simulink model "single_phase_deneme"  (R2018a)
settings: Solver=FixedStepDiscrete  StartTime=0.0  StopTime=0.07  FixedStep=5e-6  RelTol=1e-4  EnableMultiTasking=on
PreLoadFcn:
  | Ts=5e-6;
InitFcn:
  | Ts=5e-6;
libraries: powerlib x18, powerlib_meascontrol x2
Description:
  | Copyright 2008-2018 The MathWorks, Inc.
settings Model: Creator=MathWorks  LastModifiedBy=enes_
settings SolverCC: SolverResetMethod=Robust
settings DataIOCC: SaveOutput=off  SignalLogging=off  DSMLogging=off  SaveTime=off
settings OptimizationCC: LifeSpan=inf
settings DebuggingCC: ReadBeforeWriteMsg=DisableAll  WriteAfterWriteMsg=DisableAll  WriteAfterReadMsg=DisableAll  MultiTaskDSMMsg=none  SFUnexpectedBacktrackingDiag=warning  SFNoUnconditionalDefaultTransitionDiag=warning  SFExecutionAtInitializationDiag=none
settings ModelReferenceCC: UpdateModelReferenceTargets=IfOutOfDate
settings SFSimCC: SFSimEcho=off
settings CodeAppCC: StateflowObjectComments=on
settings GRTTargetCC: TargetLangStandard=C89/C90 (ANSI)  GeneratePreprocessorConditionals=Disable all
settings ConfigComp: CovMetricSettings=dw  CovHtmlReporting=on  CovSaveCumulativeToWorkspaceVar=on  CovSaveSingleToWorkspaceVar=on  CovExternalEMLEnable=off
settings SimscapeCC: SimscapeNormalizeSystem=off  SimscapeNominalValues={1, 'bar'; 1, 'cm^3/s'; 1, 'bar*kg/s'; 1, 'kJ/kg'; 1, 'kW'; }

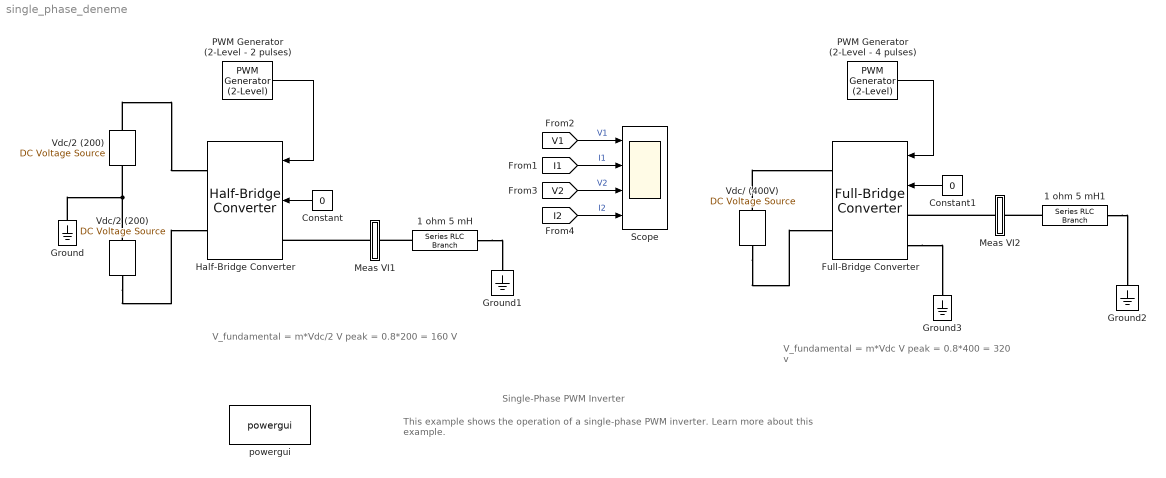
== system single_phase_deneme ==
  note: V_fundamental = m*Vdc/2 V peak
      | = 0.8*200
      | = 160 V
  note: Single-Phase PWM Inverter
  note: This example shows the operation of a single-phase PWM inverter.
      |
      | Learn more about this example.
  note: V_fundamental = m*Vdc V peak
      | = 0.8*400
      | = 320 v
  1 ohm 5 mH : powerlib/Elements/Series RLC Branch  LConnTagsString=__new0  RConnTagsString=__new0  BranchType=RL  Resistance=1  Inductance=5e-3  SetiL0=off  InitialCurrent=0  Capacitance=400e-6  Setx0=off  InitialVoltage=0  Measurements=None
  1 ohm 5 mH1 : powerlib/Elements/Series RLC Branch  LConnTagsString=__new0  RConnTagsString=__new0  BranchType=RL  Resistance=1  Inductance=5e-3  SetiL0=off  InitialCurrent=0  Capacitance=400e-6  Setx0=off  InitialVoltage=0  Measurements=None
  Constant : Constant  Value=0
  Constant1 : Constant  Value=0
  Full-Bridge Converter : powerlib/Power Electronics/Full-Bridge Converter  ModelType=Switching devices  Ron=1e-3  Rs=1e6  Cs=inf  Vforward=[0,0]  Ron_Diode=1e-3  Rs_Diode=1e6  Cs_Diode=inf  Vf_Diode=1e-3  Rs_CurrentSource=inf
      settings: SourceProductName=Simscape Power Systems  SourceProductBaseCode=PS
  Ground{,1..3} (4 alike) : powerlib/Elements/Ground  LConnTagsString=a
  Half-Bridge Converter : powerlib/Power Electronics/Half-Bridge Converter  ModelType=Switching devices  Ron=1e-3  Rs=1e6  Cs=inf  Vforward=[0,0]  Ron_Diode=1e-3  Rs_Diode=1e6  Cs_Diode=inf  Vf_Diode=1e-3  Rs_CurrentSource=inf
      settings: SourceProductName=Simscape Power Systems  SourceProductBaseCode=PS
  Meas VI1 : Subsystem
  Meas VI2 : Subsystem
  PWM Generator (2-Level - 2 pulses) : powerlib_meascontrol/Pulse & Signal Generators/PWM Generator (2-Level)  ModulatorType=Single-phase half-bridge (2 pulses)  ModulatorMode=Unsynchronized  Fc=27*60  Pc=90  nF=27  MinMax="[ -1  1 ]"  SamplingTechnique=Natural  ModulatingSignals=on  m=0.8  Freq=60  Phase=0  Ts=5e-6  ShowCarrierOutport=off
      settings: SourceProductName=Simscape Power Systems
  PWM Generator (2-Level - 4 pulses) : powerlib_meascontrol/Pulse & Signal Generators/PWM Generator (2-Level)  ModulatorType=Single-phase full-bridge (4 pulses)  ModulatorMode=Unsynchronized  Fc=27*60  Pc=90  nF=27  MinMax="[ -1  1 ]"  SamplingTechnique=Natural  ModulatingSignals=on  m=0.8  Freq=60  Phase=0  Ts=5e-6  ShowCarrierOutport=off
      settings: SourceProductName=Simscape Power Systems
  Scope : Scope  NumInputPorts=4
  Vdc/ (400V) : powerlib/Electrical Sources/DC Voltage Source  Amplitude=400  Measurements=None
  Vdc/2 (200) : powerlib/Electrical Sources/DC Voltage Source  Amplitude=200  Measurements=None
  "Vdc/2 (200) " : powerlib/Electrical Sources/DC Voltage Source  Amplitude=200  Measurements=None
  powergui : powerlib/powergui  Priority=1  SimulationMode=Discrete  SampleTime=5e-6  frequency=60  Iterations=50  frequencyindice=0  Pbase=100e6  ErrMax=1e-4  UnitsV=kV  UnitsW=MW  buscounter=0  FunctionMessages=off  echomessages=off  EnableUseOfTLC=off  CurrentSourceSwitches=off  DisableSnubberDevices=off  DisableRonSwitches=off  DisableVfSwitches=off  DisplayEquations=off  SolverType=Tustin/Backward Euler (TBE)  Interpol=off  ExternalGateDelay=off  methode=off  Ts=100  x0status=blocks  SPID=off  SwTol=0  HookPort=off  RestoreLinks=warning  ResistiveCurrentMeasurement=off  Frange=[0:2:500]  Ylog=off  Xlog=on  ShowGrid=off  save=off  variable=ZData  structure=ScopeDataForFFT  ZoomFFT=off  StartTime=0.07-2/60  cycles=2  DisplayStyle=1  fundamental=60  FreqAxis=off  MaxFrequency=5000  frequencyindicesteady=1  RmsSteady=1  display=off
  wires:
  [V1] -> Scope/1  "V1"
  PWM Generator (2-Level - 2 pulses)/1 -> Half-Bridge Converter/1
  Constant/1 -> Half-Bridge Converter/2
  PWM Generator (2-Level - 4 pulses)/1 -> Full-Bridge Converter/1
  Constant1/1 -> Full-Bridge Converter/2
  [V2] -> Scope/3  "V2"
  [I2] -> Scope/4  "I2"
  [I1] -> Scope/2  "I1"
  connections:
  Vdc/2 (200)/RConn1 -- Ground/LConn1 -- "Vdc/2 (200) "/LConn1
  "Vdc/2 (200) "/RConn1 -- Half-Bridge Converter/RConn1
  Vdc/2 (200)/LConn1 -- Half-Bridge Converter/RConn2
  Meas VI1/LConn1 -- Half-Bridge Converter/LConn1
  1 ohm 5 mH/LConn1 -- Meas VI1/RConn1
  1 ohm 5 mH/RConn1 -- Ground1/LConn1
  Meas VI2/LConn1 -- Full-Bridge Converter/LConn1
  1 ohm 5 mH1/RConn1 -- Ground2/LConn1
  1 ohm 5 mH1/LConn1 -- Meas VI2/RConn1
  Vdc/ (400V)/RConn1 -- Full-Bridge Converter/RConn1
  Vdc/ (400V)/LConn1 -- Full-Bridge Converter/RConn2
  Full-Bridge Converter/LConn2 -- Ground3/LConn1

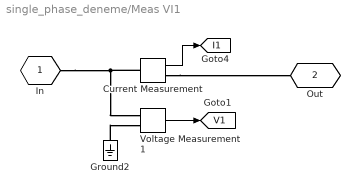
== system single_phase_deneme/Meas VI1 ==
  Current Measurement : powerlib/Measurements/Current Measurement  PhasorSimulation=off  OutputType=Complex  PSBequivalent=0
  Ground2 : powerlib/Elements/Ground  LConnTagsString=a
  Voltage Measurement1 : powerlib/Measurements/Voltage Measurement  Tag=PoWeRsYsTeMmEaSuReMeNt  PhasorSimulation=off  OutputType=Magnitude  PSBequivalent=0
  In : PMIOPort  Tag=PMCPort  Side=Left
  Out : PMIOPort  Tag=PMCPort  Port=2  Side=Right
  tag scope: I1=global, V1=global
  wires:
  Current Measurement/1 -> [I1]
  Voltage Measurement1/1 -> [V1]
  connections:
  Ground2/LConn1 -- Voltage Measurement1/LConn2
  In/RConn1 -- Current Measurement/LConn1 -- Voltage Measurement1/LConn1
  Current Measurement/RConn1 -- Out/RConn1

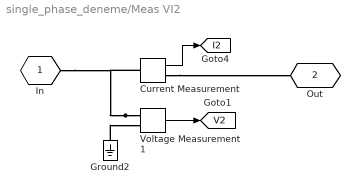
== system single_phase_deneme/Meas VI2 ==
  Current Measurement : powerlib/Measurements/Current Measurement  PhasorSimulation=off  OutputType=Complex  PSBequivalent=0
  Ground2 : powerlib/Elements/Ground  LConnTagsString=a
  Voltage Measurement1 : powerlib/Measurements/Voltage Measurement  Tag=PoWeRsYsTeMmEaSuReMeNt  PhasorSimulation=off  OutputType=Magnitude  PSBequivalent=0
  In : PMIOPort  Tag=PMCPort  Side=Left
  Out : PMIOPort  Tag=PMCPort  Port=2  Side=Right
  tag scope: I2=global, V2=global
  wires:
  Voltage Measurement1/1 -> [V2]
  Current Measurement/1 -> [I2]
  connections:
  Current Measurement/RConn1 -- Out/RConn1
  Voltage Measurement1/LConn1 -- Current Measurement/LConn1 -- In/RConn1
  Ground2/LConn1 -- Voltage Measurement1/LConn2
